simulink library "ESTS_TFY_LatForceFromFx"  (R2022a)
settings: Solver=VariableStepAuto  StartTime=0.0  StopTime=10.0  RelTol=1e-3
settings Model: Creator=blatak  LastModifiedBy=blatak

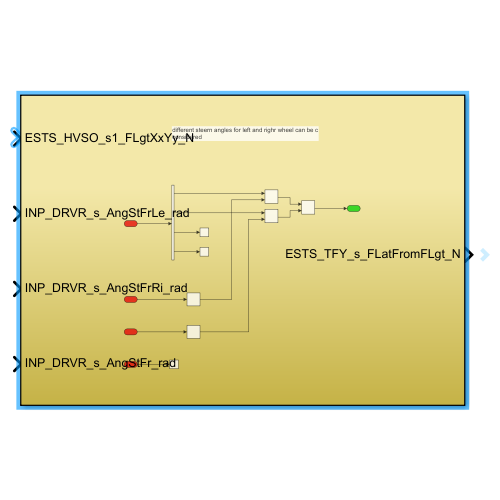
[thumbnail: Simulink's stored preview of the top-level diagram]
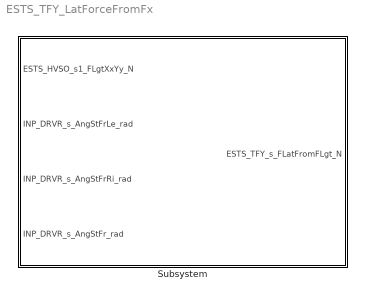
== system ESTS_TFY_LatForceFromFx ==
  Subsystem : Subsystem

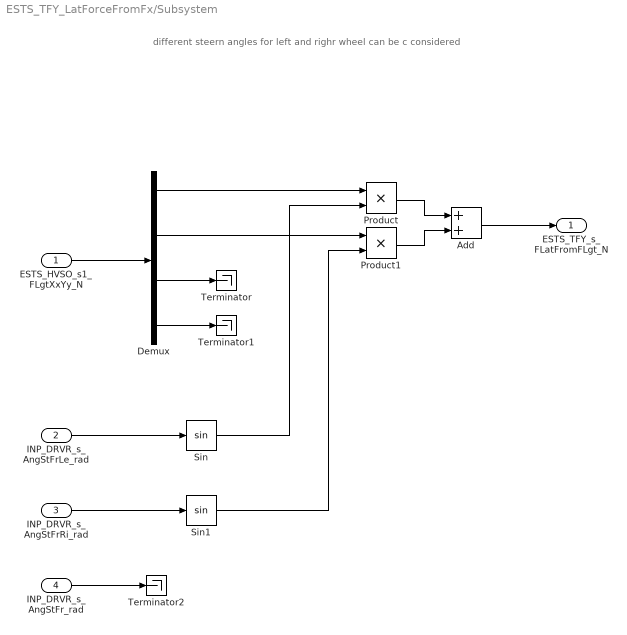
== system ESTS_TFY_LatForceFromFx/Subsystem ==
  note: different steern angles for left and righr wheel can be c
      | considered
  ESTS_HVSO_s1_FLgtXxYy_N : Inport
  INP_DRVR_s_AngStFrLe_rad : Inport  Port=2
  INP_DRVR_s_AngStFrRi_rad : Inport  Port=3
  INP_DRVR_s_AngStFr_rad : Inport  Port=4
  Add : Sum
  Demux : Demux
  Product : Product
  Product1 : Product
  Sin : Trigonometry
  Sin1 : Trigonometry
  Terminator : Terminator
  Terminator1 : Terminator
  Terminator2 : Terminator
  ESTS_TFY_s_FLatFromFLgt_N : Outport
  wires:
  Demux/2 -> Product1/1
  ESTS_HVSO_s1_FLgtXxYy_N/1 -> Demux/1
  Demux/1 -> Product/1
  Demux/4 -> Terminator1/1
  Demux/3 -> Terminator/1
  INP_DRVR_s_AngStFrLe_rad/1 -> Sin/1
  INP_DRVR_s_AngStFrRi_rad/1 -> Sin1/1
  Sin/1 -> Product/2
  Sin1/1 -> Product1/2
  Product/1 -> Add/1
  Product1/1 -> Add/2
  INP_DRVR_s_AngStFr_rad/1 -> Terminator2/1
  Add/1 -> ESTS_TFY_s_FLatFromFLgt_N/1
